simulink model "Simulations"  (R2020b)
settings: Solver=VariableStepAuto  StartTime=0.0  StopTime=100  MinStep=0.0001  RelTol=1e-3
undefined symbols (not defined in the file or in its folder): chassis, FTP, powertrain, sigbuilder_block
libraries: sdl_lib x364, nesl_utility x336, fl_lib x224, aerolibconvert2 x28, pid_lib x27
(part 1 of 15)
settings Model: Creator=moizk  LastModifiedBy=prshe

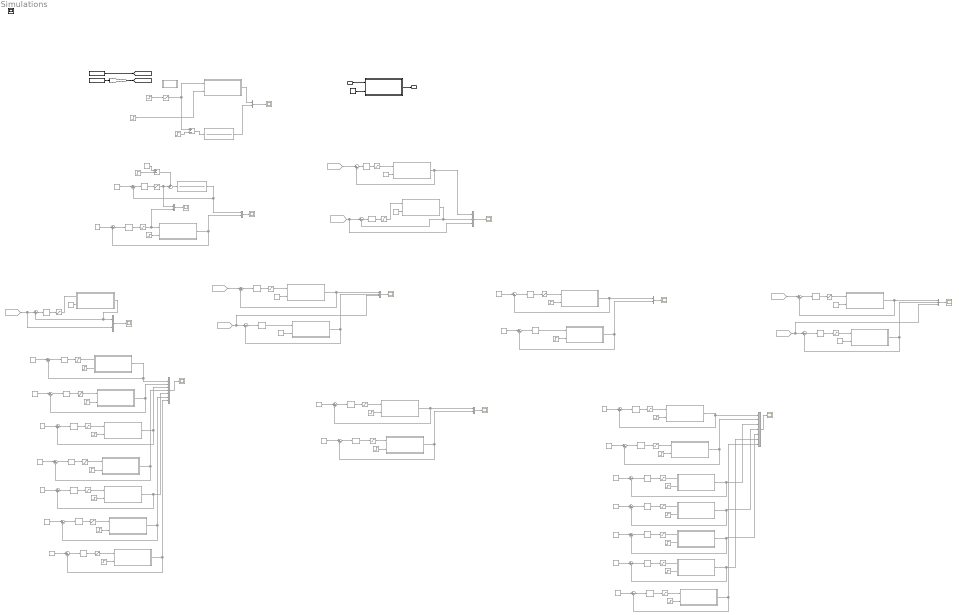
== system Simulations ==
  note: Non linear vs linear for constant speed
  note: System to linearize at a set point of 10 m/s
  note: Effect of motor delay removal on FTP
  note: Saturation block effects on FTP cycle
  note: Response to FTP
  note: Response to different hill slopes
  note: Vehicle Model
  note: Workspace (Import FTP drive cycle)
  note: Anti windup effects on constant speed with disturbance
  note: Saturation block effects on constant speed with disturbance
  note: Effects of different vehicle mass
  note: Effects of different vehicle mass for FTP
  torque : Inport
  Constant{,3..5,15..18} (8 alike) : Constant  Commented=on  Value=0
  Constant{1..2,7..14,19..28} (20 alike) : Constant  Commented=on  Value=10
  Constant6 : Constant  Value=0
  From{,1..6} (7 alike) : From  Commented=on  GotoTag=sch_cycle
  Motor removed : Subsystem  Commented=on
  Mux{,1..3,7..8} (6 alike) : Mux  Commented=on  Inputs=2
  Mux10 : Mux  Commented=on  Inputs=3
  Mux4 : Mux  Commented=on  Inputs=3
  Mux5 : Mux  Commented=on  Inputs=3
  Mux6 : Mux  Commented=on  Inputs=7
  Mux9 : Mux  Commented=on  Inputs=7
  PID Controller{1..10,12..27} (26 alike) : pid_lib/PID Controller  Commented=on  Controller=PID  Form=Parallel  TimeDomain=Continuous-time  UseExternalTs=off  SampleTime=-1  IntegratorMethod=Forward Euler  FilterMethod=Forward Euler  ControllerParametersSource=internal  P=0.8101  I=0.2270  D=0.2498  UseFilter=on  N=1000  TunerSelectOption=Transfer Function Based (PID Tuner App)  InitialConditionSource=internal  InitialConditionForIntegrator=0  InitialConditionForFilter=0  DifferentiatorICPrevScaledInput=0  ExternalReset=none  TrackingMode=off  Kt=1  LimitOutput=on  SatLimitsSource=internal  UpperSaturationLimit=powertrain.UpperTorqueLim  LowerSaturationLimit=powertrain.LowerTorqueLim  LinearizeAsGain=on  AntiWindupMode=back-calculation  Kb=0.3  POutMin=[]  POutMax=[]  IOutMin=[]  IOutMax=[]  DOutMin=[]  DOutMax=[]  NOutMin=[]  NOutMax=[]  SumOutMin=[]  SumOutMax=[]  SaturationOutMin=[]  SaturationOutMax=[]  PParamMin=[]  PParamMax=[]  IParamMin=[]  IParamMax=[]  DParamMin=[]  DParamMax=[]  NParamMin=[]  NParamMax=[]  KbParamMin=[]  KbParamMax=[]  KtParamMin=[]  KtParamMax=[]  KbOutMin=[]  KbOutMax=[]  KtOutMin=[]  KtOutMax=[]  IntegratorOutMin=[]  IntegratorOutMax=[]  FilterOutMin=[]  FilterOutMax=[]  SumI1OutMin=[]  SumI1OutMax=[]  SumI2OutMin=[]  SumI2OutMax=[]  SumI3OutMin=[]  SumI3OutMax=[]  SumI4OutMin=[]  SumI4OutMax=[]  SumDOutMin=[]  SumDOutMax=[]  DifferentiatorOutMin=[]  DifferentiatorOutMax=[]  FilterDiffOutCoefMin=[]  FilterDiffOutCoefMax=[]  ReciprocalOutMin=[]  ReciprocalOutMax=[]  SumDenOutMin=[]  SumDenOutMax=[]  SumNumOutMin=[]  SumNumOutMax=[]  DivideOutMin=[]  DivideOutMax=[]  UdiffTsProdOutMin=[]  UdiffTsProdOutMax=[]  NTsProdOutMin=[]  NTsProdOutMax=[]  UintegralTsProdOutMin=[]  UintegralTsProdOutMax=[]  UngainTsProdOutMin=[]  UngainTsProdOutMax=[]  IntegratorContinuousStateAttributes=''  IntegratorStateMustResolveToSignalObject=off  IntegratorRTWStateStorageClass=Auto  FilterContinuousStateAttributes=''  FilterStateMustResolveToSignalObject=off  FilterRTWStateStorageClass=Auto  ParallelPVariant=InternalParameters  IdealPVariant=Disabled  IVariant=InternalParameters  DVariant=InternalParameters  IntegratorVariant=Continuous  SatVariant=Enabled  AWVariant=BackCalculation  PCopyVariant=Disabled  TRVariant=Disabled  FdbkBlocksVariant=Forward  IdealPFdbkVariant=Disabled  SatFdbkVariant=Disabled  DerivativeFilterVariant=ContFilter  NVariant=InternalParameters  NCopyVariant=Disabled  FilterICVariant=InternalICsFilter  IntegratorICVariant=InternalICs  ExternalResetVariant=Disabled  TRSumVariant=Passthrough  SumFdbkVariant=Disabled  SumVariant=Sum_PID  TsampFilterVariant=InternalTs  TsampNgainVariant=Passthrough  TsampIntegralVariant=Passthrough  ExternalSaturationOutDataTypeStr=Inherit: Same as second input
  PID Controller11 : pid_lib/PID Controller  Commented=on  Controller=PID  Form=Parallel  TimeDomain=Continuous-time  UseExternalTs=off  SampleTime=-1  IntegratorMethod=Forward Euler  FilterMethod=Forward Euler  ControllerParametersSource=internal  P=0.8101  I=0.2270  D=0.2498  UseFilter=on  N=1000  TunerSelectOption=Transfer Function Based (PID Tuner App)  InitialConditionSource=internal  InitialConditionForIntegrator=0  InitialConditionForFilter=0  DifferentiatorICPrevScaledInput=0  ExternalReset=none  TrackingMode=off  Kt=1  LimitOutput=off  SatLimitsSource=internal  UpperSaturationLimit=powertrain.UpperTorqueLim  LowerSaturationLimit=powertrain.LowerTorqueLim  LinearizeAsGain=on  AntiWindupMode=back-calculation  Kb=0.3  POutMin=[]  POutMax=[]  IOutMin=[]  IOutMax=[]  DOutMin=[]  DOutMax=[]  NOutMin=[]  NOutMax=[]  SumOutMin=[]  SumOutMax=[]  SaturationOutMin=[]  SaturationOutMax=[]  PParamMin=[]  PParamMax=[]  IParamMin=[]  IParamMax=[]  DParamMin=[]  DParamMax=[]  NParamMin=[]  NParamMax=[]  KbParamMin=[]  KbParamMax=[]  KtParamMin=[]  KtParamMax=[]  KbOutMin=[]  KbOutMax=[]  KtOutMin=[]  KtOutMax=[]  IntegratorOutMin=[]  IntegratorOutMax=[]  FilterOutMin=[]  FilterOutMax=[]  SumI1OutMin=[]  SumI1OutMax=[]  SumI2OutMin=[]  SumI2OutMax=[]  SumI3OutMin=[]  SumI3OutMax=[]  SumI4OutMin=[]  SumI4OutMax=[]  SumDOutMin=[]  SumDOutMax=[]  DifferentiatorOutMin=[]  DifferentiatorOutMax=[]  FilterDiffOutCoefMin=[]  FilterDiffOutCoefMax=[]  ReciprocalOutMin=[]  ReciprocalOutMax=[]  SumDenOutMin=[]  SumDenOutMax=[]  SumNumOutMin=[]  SumNumOutMax=[]  DivideOutMin=[]  DivideOutMax=[]  UdiffTsProdOutMin=[]  UdiffTsProdOutMax=[]  NTsProdOutMin=[]  NTsProdOutMax=[]  UintegralTsProdOutMin=[]  UintegralTsProdOutMax=[]  UngainTsProdOutMin=[]  UngainTsProdOutMax=[]  IntegratorContinuousStateAttributes=''  IntegratorStateMustResolveToSignalObject=off  IntegratorRTWStateStorageClass=Auto  FilterContinuousStateAttributes=''  FilterStateMustResolveToSignalObject=off  FilterRTWStateStorageClass=Auto  ParallelPVariant=InternalParameters  IdealPVariant=Disabled  IVariant=InternalParameters  DVariant=InternalParameters  IntegratorVariant=Continuous  SatVariant=Disabled  AWVariant=Passthrough  PCopyVariant=Disabled  TRVariant=Disabled  FdbkBlocksVariant=Forward  IdealPFdbkVariant=Disabled  SatFdbkVariant=Disabled  DerivativeFilterVariant=ContFilter  NVariant=InternalParameters  NCopyVariant=Disabled  FilterICVariant=InternalICsFilter  IntegratorICVariant=InternalICs  ExternalResetVariant=Disabled  TRSumVariant=Passthrough  SumFdbkVariant=Disabled  SumVariant=Sum_PID  TsampFilterVariant=InternalTs  TsampNgainVariant=Passthrough  TsampIntegralVariant=Passthrough  ExternalSaturationOutDataTypeStr=Inherit: Same as second input
  Plant Model : Subsystem  Commented=on
  Plant Model1 : Subsystem
  Plant Model10 : Subsystem  Commented=on
  Plant Model11 : Subsystem  Commented=on
  Plant Model12 : Subsystem  Commented=on
  Plant Model13 : Subsystem  Commented=on
  Plant Model14 : Subsystem  Commented=on
  Plant Model15 : Subsystem  Commented=on
  Plant Model16 : Subsystem  Commented=on
  Plant Model17 : Subsystem  Commented=on
  Plant Model18 : Subsystem  Commented=on
  Plant Model19 : Subsystem  Commented=on
  Plant Model2 : Subsystem  Commented=on
  Plant Model20 : Subsystem  Commented=on
  Plant Model21 : Subsystem  Commented=on
  Plant Model22 : Subsystem  Commented=on
  Plant Model23 : Subsystem  Commented=on
  Plant Model24 : Subsystem  Commented=on
  Plant Model25 : Subsystem  Commented=on
  Plant Model26 : Subsystem  Commented=on
  Plant Model3 : Subsystem  Commented=on
  Plant Model4 : Subsystem  Commented=on
  Plant Model5 : Subsystem  Commented=on
  Plant Model6 : Subsystem  Commented=on
  Plant Model7 : Subsystem  Commented=on
  Plant Model8 : Subsystem  Commented=on
  Plant Model9 : Subsystem  Commented=on
  Saturation{1..26} (26 alike) : Saturate  Commented=on  UpperLimit=powertrain.UpperTorqueLim  LowerLimit=powertrain.LowerTorqueLim
  Scale Trace Spd : Gain  Gain=FTP.ScaledSpd
  Scope{,3..4,7..14} (11 alike) : Scope  Commented=on
  Step : Step  Commented=on  After=0.6484  SampleTime=0
  Step{1,3,5..6,8..12,18..22} (14 alike) : Step  Commented=on  Time=50  After=4  SampleTime=0
  Step13 : Step  Commented=on  Time=50  After=6  SampleTime=0
  Step14 : Step  Commented=on  Time=50  After=7  SampleTime=0
  Step15 : Step  Commented=on  Time=50  After=8  SampleTime=0
  Step16 : Step  Commented=on  Time=50  After=9  SampleTime=0
  Step17 : Step  Commented=on  Time=50  After=10  SampleTime=0
  Step2 : Step  Commented=on  Time=50  After=0.1987  SampleTime=0
  Step4 : Step  Commented=on  Time=50  After=0.1987  SampleTime=0
  Step7 : Step  Commented=on  Time=50  After=5  SampleTime=0
  Subtract : Sum  Commented=on  Inputs=+-
  Subtract1 : Sum  Commented=on  Inputs=+-
  Sum{,2..27} (27 alike) : Sum  Commented=on  Inputs=|+-
  Sum1 : Sum  Commented=on  Inputs=++|
  Transfer Fcn : TransferFcn  Commented=on  Numerator=[67.24]  Denominator=[1 12.22 22.63 4.36]
  Transfer Fcn2 : TransferFcn  Commented=on  Numerator=[67.24]  Denominator=[1 12.22 22.63 4.36]
  WrkSp Road Slope (Zero) : FromWorkspace  VariableName=FTP.sch_grade.data
  Wrksp Drive Cycle : FromWorkspace  VariableName=FTP.sch_cycle.data
  trq_cmd4 : Subsystem  Tag=STV Subsys  Commented=on  LoadFcn=sigbuilder_block('load');  StartFcn=sigbuilder_block('start');  StopFcn=sigbuilder_block('stop');  ClipboardFcn=sigbuilder_block('clipboard');  mask(Sigbuilder block){tuvar=[0:10]}
      mask help: Simulink:masks:SigbuilderBlock_MD
      mask init:
      | if ~strcmp(get_param(bdroot(gcbh),'SimulationStatus'),'stopped') tuvar = sigbuilder_block('maskInit'); end
      settings: CopyFcn=sigbuilder_block('copy');  DeleteFcn=sigbuilder_block('delete');  ModelCloseFcn=sigbuilder_block('modelClose');  PreSaveFcn=sigbuilder_block('preSave');  PauseFcn=sigbuilder_block('pause');  ContinueFcn=sigbuilder_block('continue');  NameChangeFcn=sigbuilder_block('namechange');  OpenFcn=sigbuilder_block('open',[0 30 1152 561.6 ]);  CloseFcn=sigbuilder_block('close');
      mask Display: plot(0, 0, 100, 100,[2, 2, 32, 32, 2], [68, 8, 8, 68, 68],[32, 2], [38, 38], [32, 19, 2],[53, 60, 44], [32, 17, 17, 2],[16, 16, 31, 31]);txt = getActiveGroup(gcbh);text(2, 100, txt,'verticalAlignment', 'top');
  speed : Outport
  Scope{1..2,5..6} (4 alike) : Scope
  wires:
  WrkSp Road Slope (Zero)/1 -> [sch_grade]
  Step1/1 -> Plant Model/2(road_grade)
  Plant Model/1(veh_spd_lin) -> Mux/1  "Model Velo (m/s)"
  Wrksp Drive Cycle/1 -> Scale Trace Spd/1
  Scale Trace Spd/1 -> [sch_cycle]
  Step/1 -> Saturation1/1  "trq_cmd"
  Saturation1/1 -> Subtract/1, Plant Model/1(trq_cmd)  "trq_act"
  Mux/1 -> Scope/1
  Transfer Fcn/1 -> Mux/2
  Step2/1 -> Subtract/2
  Subtract/1 -> Transfer Fcn/1
  Plant Model3/1(veh_spd_lin) -> Mux1/1, Sum/2  "Output Speed"
  Sum/1 -> PID Controller2/1
  From/1 -> Mux1/2, Sum/1  "Desired Speed"
  Step4/1 -> Subtract1/2
  Constant/1 -> Subtract1/1
  PID Controller2/1 -> Saturation2/1
  Saturation2/1 -> Plant Model3/1(trq_cmd)
  Mux1/1 -> Scope3/1
  Sum1/1 -> Transfer Fcn2/1
  Transfer Fcn2/1 -> Mux2/1, Sum2/2  "Linear"
  PID Controller10/1 -> Saturation3/1  "before sat"
  Saturation3/1 -> Mux3/1, Sum1/2  "torque-linear"
  Subtract1/1 -> Sum1/1
  Constant2/1 -> Sum2/1
  Sum2/1 -> PID Controller10/1
  Constant6/1 -> Plant Model1/2(road_grade)
  torque/1 -> Plant Model1/1(trq_cmd)
  Plant Model1/1(veh_spd_lin) -> speed/1
  PID Controller1/1 -> Saturation4/1
  Sum4/1 -> PID Controller1/1
  Plant Model2/1(veh_spd_lin) -> Mux2/2, Sum4/2  "Nonlinear"
  Constant1/1 -> Sum4/1
  Saturation4/1 -> Mux3/2, Plant Model2/1(trq_cmd)  "torque-nonlinear"
  Step6/1 -> Plant Model2/2(road_grade)
  Mux2/1 -> Scope4/1
  Mux3/1 -> Scope7/1
  Constant3/1 -> Plant Model3/2(road_grade)
  Constant4/1 -> Plant Model4/2(road_grade)
  PID Controller4/1 -> Saturation5/1
  Saturation5/1 -> Plant Model4/1(trq_cmd)
  Mux4/1 -> Scope8/1
  Plant Model4/1(veh_spd_lin) -> Sum3/2, Mux4/2  "Control"
  Sum3/1 -> PID Controller4/1
  From1/1 -> Mux4/3, Sum3/1  "Desired Speed"
  From2/1 -> Sum5/1  "Desired Speed"
  Sum5/1 -> PID Controller3/1
  PID Controller3/1 -> Saturation6/1
  Saturation6/1 -> Motor removed/1(trq_cmd)
  Constant5/1 -> Motor removed/2(road_grade)
  Motor removed/1(veh_spd_lin) -> Mux4/1, Sum5/2  "Motor removed"
  From3/1 -> Sum6/1
  Constant15/1 -> Plant Model5/2(road_grade)
  Plant Model5/1(veh_spd_lin) -> Mux5/1, Sum6/2  "Saturation"
  PID Controller5/1 -> Saturation7/1
  Sum6/1 -> PID Controller5/1
  Saturation7/1 -> Plant Model5/1(trq_cmd)  "torque-nonlinear"
  From4/1 -> Mux5/3, Sum7/1  "Desired Speed"
  Constant16/1 -> Plant Model6/2(road_grade)
  Plant Model6/1(veh_spd_lin) -> Mux5/2, Sum7/2  "No saturation"
  Sum7/1 -> PID Controller6/1
  PID Controller6/1 -> Plant Model6/1(trq_cmd)  "torque-nonlinear"
  Mux5/1 -> Scope9/1
  Constant9/1 -> Sum8/1
  Step7/1 -> Plant Model7/2(road_grade)
  Plant Model7/1(veh_spd_lin) -> Mux6/2, Sum8/2  "5 degrees"
  PID Controller8/1 -> Saturation8/1
  Sum8/1 -> PID Controller8/1
  Saturation8/1 -> Plant Model7/1(trq_cmd)  "torque-nonlinear"
  Sum9/1 -> PID Controller7/1
  Plant Model8/1(veh_spd_lin) -> Mux6/1, Sum9/2  "4 degrees"
  Step8/1 -> Plant Model8/2(road_grade)
  PID Controller7/1 -> Saturation9/1
  Saturation9/1 -> Plant Model8/1(trq_cmd)  "torque-nonlinear"
  Constant10/1 -> Sum9/1
  Mux6/1 -> Scope10/1
  Mux7/1 -> Scope11/1
  Saturation10/1 -> Plant Model9/1(trq_cmd)  "torque-nonlinear"
  Plant Model9/1(veh_spd_lin) -> Mux7/1, Sum10/2  "With anti-windup"
  Step9/1 -> Plant Model9/2(road_grade)
  Constant11/1 -> Sum10/1
  Sum10/1 -> PID Controller9/1
  PID Controller11/1 -> Saturation11/1  "torque-nonlinear"
  Sum11/1 -> PID Controller11/1
  PID Controller9/1 -> Saturation10/1
  Plant Model10/1(veh_spd_lin) -> Mux7/2, Sum11/2  "No anti-windup"
  Constant12/1 -> Sum11/1
  Step10/1 -> Plant Model10/2(road_grade)
  Saturation11/1 -> Plant Model10/1(trq_cmd)  "torque-nonlinear"
  Mux8/1 -> Scope12/1
  Saturation12/1 -> Plant Model11/1(trq_cmd)  "torque-nonlinear"
  Plant Model11/1(veh_spd_lin) -> Mux8/1, Sum12/2  "Saturation"
  Step11/1 -> Plant Model11/2(road_grade)
  Constant13/1 -> Sum12/1
  Sum12/1 -> PID Controller12/1
  PID Controller13/1 -> Plant Model12/1(trq_cmd)  "torque-nonlinear"
  Sum13/1 -> PID Controller13/1
  PID Controller12/1 -> Saturation12/1
  Plant Model12/1(veh_spd_lin) -> Mux8/2, Sum13/2  "No saturation"
  Constant14/1 -> Sum13/1
  Step12/1 -> Plant Model12/2(road_grade)
  Sum15/1 -> PID Controller15/1
  Constant8/1 -> Sum15/1
  Plant Model14/1(veh_spd_lin) -> Sum15/2, Mux9/2  "5kg"
  Step5/1 -> Plant Model14/2(road_grade)
  PID Controller14/1 -> Saturation13/1
  Sum14/1 -> PID Controller14/1
  PID Controller15/1 -> Saturation14/1  "torque-nonlinear"
  Constant7/1 -> Sum14/1
  Mux9/1 -> Scope13/1
  Plant Model13/1(veh_spd_lin) -> Sum14/2, Mux9/1  "4.84kg"
  Saturation13/1 -> Plant Model13/1(trq_cmd)  "torque-nonlinear"
  Step3/1 -> Plant Model13/2(road_grade)
  Saturation14/1 -> Plant Model14/1(trq_cmd)  "torque-nonlinear"
  Sum16/1 -> PID Controller16/1
  Saturation16/1 -> Plant Model16/1(trq_cmd)  "torque-nonlinear"
  PID Controller16/1 -> Saturation15/1
  PID Controller17/1 -> Saturation16/1  "torque-nonlinear"
  Constant18/1 -> Plant Model16/2(road_grade)
  Plant Model16/1(veh_spd_lin) -> Mux10/2, Sum17/2  "6kg"
  From5/1 -> Sum16/1
  Sum17/1 -> PID Controller17/1
  Mux10/1 -> Scope14/1
  Plant Model15/1(veh_spd_lin) -> Mux10/1, Sum16/2  "4.84kg"
  Constant17/1 -> Plant Model15/2(road_grade)
  Saturation15/1 -> Plant Model15/1(trq_cmd)  "torque-nonlinear"
  From6/1 -> Mux10/3, Sum17/1  "Desired speed"
  PID Controller18/1 -> Saturation17/1
  Plant Model17/1(veh_spd_lin) -> Mux6/3, Sum18/2  "6 degrees"
  Sum18/1 -> PID Controller18/1
  Step13/1 -> Plant Model17/2(road_grade)
  Constant19/1 -> Sum18/1
  Saturation17/1 -> Plant Model17/1(trq_cmd)  "torque-nonlinear"
  PID Controller19/1 -> Saturation18/1
  Plant Model18/1(veh_spd_lin) -> Mux6/4, Sum19/2  "7 degrees"
  Sum19/1 -> PID Controller19/1
  Step14/1 -> Plant Model18/2(road_grade)
  Constant20/1 -> Sum19/1
  Saturation18/1 -> Plant Model18/1(trq_cmd)  "torque-nonlinear"
  PID Controller20/1 -> Saturation19/1
  Plant Model19/1(veh_spd_lin) -> Mux6/5, Sum20/2  "8 degrees"
  Sum20/1 -> PID Controller20/1
  Step15/1 -> Plant Model19/2(road_grade)
  Constant21/1 -> Sum20/1
  Saturation19/1 -> Plant Model19/1(trq_cmd)  "torque-nonlinear"
  PID Controller21/1 -> Saturation20/1
  Plant Model20/1(veh_spd_lin) -> Mux6/6, Sum21/2  "9 degrees"
  Sum21/1 -> PID Controller21/1
  Step16/1 -> Plant Model20/2(road_grade)
  Constant22/1 -> Sum21/1
  Saturation20/1 -> Plant Model20/1(trq_cmd)  "torque-nonlinear"
  PID Controller22/1 -> Saturation21/1
  Plant Model21/1(veh_spd_lin) -> Mux6/7, Sum22/2  "10 degrees"
  Sum22/1 -> PID Controller22/1
  Step17/1 -> Plant Model21/2(road_grade)
  Constant23/1 -> Sum22/1
  Saturation21/1 -> Plant Model21/1(trq_cmd)  "torque-nonlinear"
  Plant Model22/1(veh_spd_lin) -> Mux9/3, Sum23/2  "6kg"
  Saturation22/1 -> Plant Model22/1(trq_cmd)  "torque-nonlinear"
  Sum23/1 -> PID Controller23/1
  Constant24/1 -> Sum23/1
  Step18/1 -> Plant Model22/2(road_grade)
  PID Controller23/1 -> Saturation22/1  "torque-nonlinear"
  Plant Model23/1(veh_spd_lin) -> Mux9/4, Sum24/2  "7kg"
  Saturation23/1 -> Plant Model23/1(trq_cmd)  "torque-nonlinear"
  Sum24/1 -> PID Controller24/1
  Constant25/1 -> Sum24/1
  Step19/1 -> Plant Model23/2(road_grade)
  PID Controller24/1 -> Saturation23/1  "torque-nonlinear"
  Plant Model24/1(veh_spd_lin) -> Mux9/5, Sum25/2  "8kg"
  Saturation24/1 -> Plant Model24/1(trq_cmd)  "torque-nonlinear"
  Sum25/1 -> PID Controller25/1
  Constant26/1 -> Sum25/1
  Step20/1 -> Plant Model24/2(road_grade)
  PID Controller25/1 -> Saturation24/1  "torque-nonlinear"
  Plant Model25/1(veh_spd_lin) -> Mux9/6, Sum26/2  "9kg"
  Saturation25/1 -> Plant Model25/1(trq_cmd)  "torque-nonlinear"
  Sum26/1 -> PID Controller26/1
  Constant27/1 -> Sum26/1
  Step21/1 -> Plant Model25/2(road_grade)
  PID Controller26/1 -> Saturation25/1  "torque-nonlinear"
  Plant Model26/1(veh_spd_lin) -> Mux9/7, Sum27/2  "10kg"
  Saturation26/1 -> Plant Model26/1(trq_cmd)  "torque-nonlinear"
  Sum27/1 -> PID Controller27/1
  Constant28/1 -> Sum27/1
  Step22/1 -> Plant Model26/2(road_grade)
  PID Controller27/1 -> Saturation26/1  "torque-nonlinear"

== system Simulations/Motor removed ==
  note: Chassis
  note: Motor Dynamics
  note: Drivetrain
  trq_cmd : Inport
  road_grade : Inport  Port=2
  Angle Conversion3 : aerolibconvert2/Angle Conversion  IU=deg  OU=rad
  Belt Drive FL : sdl_lib/Couplings & Drives/Belt Drive  drive_type=sdl.enum.wrap_configuration.open  belt_type=sdl.enum.belt_type.ideal  sheave_ang=30 deg  num_belts=1  model_f_c=sdl.enum.model_centrifugal.off  linear_density=0.6 kg/m  model_compliance=sdl.enum.compliance.off  stiffness=1e4 N/m  damping=1e3 N/(m/s)  tension=100 N  breakable=sdl.enum.max_tension.off  F_max=1e5 N  r_pulley_A=drivetrain.RadiusA m  r_pulley_B=drivetrain.RadiusB m  b_pulley_A=drivetrain.bvfCoeffA N*m/(rad/s)  b_pulley_B=drivetrain.bvfCoeffB N*m/(rad/s)  model_inertia_A=sdl.enum.model_inertia.off  model_inertia_B=sdl.enum.model_inertia.off  pulley_inertia_A=0.01 kg*m^2  pulley_inertia_B=0.03 kg*m^2  initial_velocity_A=0 rad/s  initial_velocity_B=0 rad/s  mu=0.5  wrap_parameterization=sdl.enum.wrap_parameterization.centers  d_centers=0.5 m  phi_wrap_A=145 deg  phi_wrap_B=215 deg  v_thr=0.001 m/s
      settings: SourceProductBaseCode=LD  InternalSimscapePortConfiguration="{\"Bottom\":[],\"Left\":[{\"id\":\"A\",\"label\":\"A\",\"type\":\"foundation.mechanical.rotational.rotational\"}],\"Right\":[{\"id\":\"B\",\"label\":\"B\",\"type\":\"foundation.mechanical.rotational.rotational\"}],\"Top\":[]}"
  Belt Drive FR : sdl_lib/Couplings & Drives/Belt Drive  drive_type=sdl.enum.wrap_configuration.open  belt_type=sdl.enum.belt_type.ideal  sheave_ang=30 deg  num_belts=1  model_f_c=sdl.enum.model_centrifugal.off  linear_density=0.6 kg/m  model_compliance=sdl.enum.compliance.off  stiffness=1e4 N/m  damping=1e3 N/(m/s)  tension=100 N  breakable=sdl.enum.max_tension.off  F_max=1e5 N  r_pulley_A=drivetrain.RadiusA m  r_pulley_B=drivetrain.RadiusB m  b_pulley_A=drivetrain.bvfCoeffA N*m/(rad/s)  b_pulley_B=drivetrain.bvfCoeffB N*m/(rad/s)  model_inertia_A=sdl.enum.model_inertia.off  model_inertia_B=sdl.enum.model_inertia.off  pulley_inertia_A=0.01 kg*m^2  pulley_inertia_B=0.03 kg*m^2  initial_velocity_A=0 rad/s  initial_velocity_B=0 rad/s  mu=0.5  wrap_parameterization=sdl.enum.wrap_parameterization.centers  d_centers=0.5 m  phi_wrap_A=145 deg  phi_wrap_B=215 deg  v_thr=0.001 m/s
      settings: SourceProductBaseCode=LD  InternalSimscapePortConfiguration="{\"Bottom\":[],\"Left\":[{\"id\":\"A\",\"label\":\"A\",\"type\":\"foundation.mechanical.rotational.rotational\"}],\"Right\":[{\"id\":\"B\",\"label\":\"B\",\"type\":\"foundation.mechanical.rotational.rotational\"}],\"Top\":[]}"
  Belt Drive RL : sdl_lib/Couplings & Drives/Belt Drive  drive_type=sdl.enum.wrap_configuration.open  belt_type=sdl.enum.belt_type.ideal  sheave_ang=30 deg  num_belts=1  model_f_c=sdl.enum.model_centrifugal.off  linear_density=0.6 kg/m  model_compliance=sdl.enum.compliance.off  stiffness=1e4 N/m  damping=1e3 N/(m/s)  tension=100 N  breakable=sdl.enum.max_tension.off  F_max=1e5 N  r_pulley_A=drivetrain.RadiusA m  r_pulley_B=drivetrain.RadiusB m  b_pulley_A=drivetrain.bvfCoeffA N*m/(rad/s)  b_pulley_B=drivetrain.bvfCoeffB N*m/(rad/s)  model_inertia_A=sdl.enum.model_inertia.off  model_inertia_B=sdl.enum.model_inertia.off  pulley_inertia_A=0.01 kg*m^2  pulley_inertia_B=0.03 kg*m^2  initial_velocity_A=0 rad/s  initial_velocity_B=0 rad/s  mu=0.5  wrap_parameterization=sdl.enum.wrap_parameterization.centers  d_centers=0.5 m  phi_wrap_A=145 deg  phi_wrap_B=215 deg  v_thr=0.001 m/s
      settings: SourceProductBaseCode=LD  InternalSimscapePortConfiguration="{\"Bottom\":[],\"Left\":[{\"id\":\"A\",\"label\":\"A\",\"type\":\"foundation.mechanical.rotational.rotational\"}],\"Right\":[{\"id\":\"B\",\"label\":\"B\",\"type\":\"foundation.mechanical.rotational.rotational\"}],\"Top\":[]}"
  Belt Drive RR : sdl_lib/Couplings & Drives/Belt Drive  drive_type=sdl.enum.wrap_configuration.open  belt_type=sdl.enum.belt_type.ideal  sheave_ang=30 deg  num_belts=1  model_f_c=sdl.enum.model_centrifugal.off  linear_density=0.6 kg/m  model_compliance=sdl.enum.compliance.off  stiffness=1e4 N/m  damping=1e3 N/(m/s)  tension=100 N  breakable=sdl.enum.max_tension.off  F_max=1e5 N  r_pulley_A=drivetrain.RadiusA m  r_pulley_B=drivetrain.RadiusB m  b_pulley_A=drivetrain.bvfCoeffA N*m/(rad/s)  b_pulley_B=drivetrain.bvfCoeffB N*m/(rad/s)  model_inertia_A=sdl.enum.model_inertia.off  model_inertia_B=sdl.enum.model_inertia.off  pulley_inertia_A=0.01 kg*m^2  pulley_inertia_B=0.03 kg*m^2  initial_velocity_A=0 rad/s  initial_velocity_B=0 rad/s  mu=0.5  wrap_parameterization=sdl.enum.wrap_parameterization.centers  d_centers=0.5 m  phi_wrap_A=145 deg  phi_wrap_B=215 deg  v_thr=0.001 m/s
      settings: SourceProductBaseCode=LD  InternalSimscapePortConfiguration="{\"Bottom\":[],\"Left\":[{\"id\":\"A\",\"label\":\"A\",\"type\":\"foundation.mechanical.rotational.rotational\"}],\"Right\":[{\"id\":\"B\",\"label\":\"B\",\"type\":\"foundation.mechanical.rotational.rotational\"}],\"Top\":[]}"
  Constant : Constant  Value=0
  Ideal Torque Source FL : fl_lib/Mechanical/Mechanical Sources/Ideal Torque Source
  Ideal Torque Source FR : fl_lib/Mechanical/Mechanical Sources/Ideal Torque Source
  Ideal Torque Source RL : fl_lib/Mechanical/Mechanical Sources/Ideal Torque Source
  Ideal Torque Source RR : fl_lib/Mechanical/Mechanical Sources/Ideal Torque Source
  Mechanical Rotational Reference{1..3,8} (4 alike) : fl_lib/Mechanical/Rotational Elements/Mechanical Rotational Reference
  PS-Simulink Converter{,1,3..4} (4 alike) : nesl_utility/PS-Simulink Converter  PhysicalDomain=network_engine_domain  SubClassName=ps_output  LeftPortType=input  RightPortType=output  PseudoPeriodic=off  Frequencies=[]  Unit=inherit  AffineConversion=off
  Simulink-PS Converter{3,9..12} (5 alike) : nesl_utility/Simulink-PS Converter  PhysicalDomain=network_engine_domain  SubClassName=ps_input  LeftPortType=input  RightPortType=output  PseudoPeriodic=off  Frequencies=[]  NoiseDistribution=none  NoiseParameters=[]  Unit=1  AffineConversion=off  FilteringAndDerivatives=provide  SimscapeFilterOrder=1  InputFilterTimeConstant=0.001  UdotUserProvided=0
  Simulink-PS Converter8 : nesl_utility/Simulink-PS Converter  PhysicalDomain=network_engine_domain  SubClassName=ps_input  LeftPortType=input  RightPortType=output  PseudoPeriodic=off  Frequencies=[]  NoiseDistribution=none  NoiseParameters=[]  Unit=rad  AffineConversion=off  FilteringAndDerivatives=provide  SimscapeFilterOrder=1  InputFilterTimeConstant=0.001  UdotUserProvided=0
  Solver Configuration2 : nesl_utility/Solver Configuration  PhysicalDomain=network_engine_domain  SubClassName=solver  LeftPortType=input  RightPortType=generic  Tones=[]  Harmonics=[]  SimulateNoise=off  Profile=off  UseLocalSampling=off  EnableSwitchedLinearOptims=on  FrequencyDomain=off  UseCCode=off  RelTol=0.001  AbsTol=1e-06  MinStep=1e-09  ToWorkspace=off  RevertToSquareIcSolve=off  NumHomotopyIterations=100  PhasorMode=off  PhasorModeNumHarmonics=1  DoDC=off  ResidualTolerance=1e-09  UseLocalSolver=off  LocalSolverChoice=NE_BACKWARD_EULER_ADVANCER  LocalSolverSampleTime=0.001  DoFixedCost=off  MaxNonlinIter=3  MaxModeIter=2  ComputeImpulses=off  ImpulseIterations=2  LinearAlgebra=auto  EquationFormulation=NE_TIME_EF  DelaysMemoryBudget=1024  AutomaticFiltering=on  FilteringTimeConstant=0.001  PartitionStorageMethod=AS_NEEDED  PartitionMemoryBudget=1024  PartitionMethod=ROBUST
  Terminator{,1..3} (4 alike) : Terminator
  Tire (Simple) FL : sdl_lib/Tires & Vehicles/Tire (Simple)  r_tire=drivetrain.RolRadius m  model_compliance=0  stiffness=1e6 N/m  damping=1000 N/(m/s)  model_inertia=0  tire_inertia=drivetrain.IyyWhl kg*m^2  initial_velocity=drivetrain.InitVelo rad/s
      settings: SourceProductBaseCode=LD  InternalSimscapePortConfiguration="{\"Bottom\":[],\"Left\":[{\"id\":\"A\",\"label\":\"A\",\"type\":\"foundation.mechanical.rotational.rotational\"}],\"Right\":[{\"id\":\"H\",\"label\":\"H\",\"type\":\"foundation.mechanical.translational.translational\"}],\"Top\":[]}"
  Tire (Simple) FR : sdl_lib/Tires & Vehicles/Tire (Simple)  r_tire=drivetrain.RolRadius m  model_compliance=0  stiffness=1e6 N/m  damping=1000 N/(m/s)  model_inertia=0  tire_inertia=drivetrain.IyyWhl kg*m^2  initial_velocity=drivetrain.InitVelo rad/s
      settings: SourceProductBaseCode=LD  InternalSimscapePortConfiguration="{\"Bottom\":[],\"Left\":[{\"id\":\"A\",\"label\":\"A\",\"type\":\"foundation.mechanical.rotational.rotational\"}],\"Right\":[{\"id\":\"H\",\"label\":\"H\",\"type\":\"foundation.mechanical.translational.translational\"}],\"Top\":[]}"
  Tire (Simple) RL : sdl_lib/Tires & Vehicles/Tire (Simple)  r_tire=drivetrain.RolRadius m  model_compliance=0  stiffness=1e6 N/m  damping=1000 N/(m/s)  model_inertia=0  tire_inertia=drivetrain.IyyWhl kg*m^2  initial_velocity=drivetrain.InitVelo rad/s
      settings: SourceProductBaseCode=LD  InternalSimscapePortConfiguration="{\"Bottom\":[],\"Left\":[{\"id\":\"A\",\"label\":\"A\",\"type\":\"foundation.mechanical.rotational.rotational\"}],\"Right\":[{\"id\":\"H\",\"label\":\"H\",\"type\":\"foundation.mechanical.translational.translational\"}],\"Top\":[]}"
  Tire (Simple) RR : sdl_lib/Tires & Vehicles/Tire (Simple)  r_tire=drivetrain.RolRadius m  model_compliance=0  stiffness=1e6 N/m  damping=1000 N/(m/s)  model_inertia=0  tire_inertia=drivetrain.IyyWhl kg*m^2  initial_velocity=drivetrain.InitVelo rad/s
      settings: SourceProductBaseCode=LD  InternalSimscapePortConfiguration="{\"Bottom\":[],\"Left\":[{\"id\":\"A\",\"label\":\"A\",\"type\":\"foundation.mechanical.rotational.rotational\"}],\"Right\":[{\"id\":\"H\",\"label\":\"H\",\"type\":\"foundation.mechanical.translational.translational\"}],\"Top\":[]}"
  Tire-Road Interaction (Magic Formula) FL : sdl_lib/Tires & Vehicles/Tire Subcomponents/Tire-Road Interaction (Magic Formula)  parameterization=sdl.enum.magic_tire_model.peak  F_z1=drivetrain.VertLoad N  F_x1=drivetrain.PeakLongF N  kappa1=drivetrain.Slip  B_m=10  C_m=1.9  D_m=1  E_m=0.97  fz0=4000 N  p_Cx=1.685  p_Dx=[1.21, -.037]  p_Ex=[.344, .095, -.02, 0]  p_Kx=[21.51, -.163, .245]  p_Hx=[-.002, .002]  p_Vx=[0, 0]  v_tr_thr=drivetrain.VeloTrhd m/s
      settings: SourceProductBaseCode=LD  InternalSimscapePortConfiguration="{\"Bottom\":[],\"Left\":[{\"id\":\"N\",\"label\":\"N\",\"type\":\"input\"},{\"id\":\"T\",\"label\":\"T\",\"type\":\"foundation.mechanical.translational.translational\"}],\"Right\":[{\"id\":\"S\",\"label\":\"S\",\"type\":\"output\"},{\"id\":\"H\",\"label\":\"H\",\"type\":\"foundation.mechanical.translational.translational\"}],\"Top\":[]}"
  Tire-Road Interaction (Magic Formula) FR : sdl_lib/Tires & Vehicles/Tire Subcomponents/Tire-Road Interaction (Magic Formula)  parameterization=sdl.enum.magic_tire_model.peak  F_z1=drivetrain.VertLoad N  F_x1=drivetrain.PeakLongF N  kappa1=drivetrain.Slip  B_m=10  C_m=1.9  D_m=1  E_m=0.97  fz0=4000 N  p_Cx=1.685  p_Dx=[1.21, -.037]  p_Ex=[.344, .095, -.02, 0]  p_Kx=[21.51, -.163, .245]  p_Hx=[-.002, .002]  p_Vx=[0, 0]  v_tr_thr=drivetrain.VeloTrhd m/s
      settings: SourceProductBaseCode=LD  InternalSimscapePortConfiguration="{\"Bottom\":[],\"Left\":[{\"id\":\"N\",\"label\":\"N\",\"type\":\"input\"},{\"id\":\"T\",\"label\":\"T\",\"type\":\"foundation.mechanical.translational.translational\"}],\"Right\":[{\"id\":\"S\",\"label\":\"S\",\"type\":\"output\"},{\"id\":\"H\",\"label\":\"H\",\"type\":\"foundation.mechanical.translational.translational\"}],\"Top\":[]}"
  Tire-Road Interaction (Magic Formula) RL : sdl_lib/Tires & Vehicles/Tire Subcomponents/Tire-Road Interaction (Magic Formula)  parameterization=sdl.enum.magic_tire_model.peak  F_z1=drivetrain.VertLoad N  F_x1=drivetrain.PeakLongF N  kappa1=drivetrain.Slip  B_m=10  C_m=1.9  D_m=1  E_m=0.97  fz0=4000 N  p_Cx=1.685  p_Dx=[1.21, -.037]  p_Ex=[.344, .095, -.02, 0]  p_Kx=[21.51, -.163, .245]  p_Hx=[-.002, .002]  p_Vx=[0, 0]  v_tr_thr=drivetrain.VeloTrhd m/s
      settings: SourceProductBaseCode=LD  InternalSimscapePortConfiguration="{\"Bottom\":[],\"Left\":[{\"id\":\"N\",\"label\":\"N\",\"type\":\"input\"},{\"id\":\"T\",\"label\":\"T\",\"type\":\"foundation.mechanical.translational.translational\"}],\"Right\":[{\"id\":\"S\",\"label\":\"S\",\"type\":\"output\"},{\"id\":\"H\",\"label\":\"H\",\"type\":\"foundation.mechanical.translational.translational\"}],\"Top\":[]}"
  Tire-Road Interaction (Magic Formula) RR : sdl_lib/Tires & Vehicles/Tire Subcomponents/Tire-Road Interaction (Magic Formula)  parameterization=sdl.enum.magic_tire_model.peak  F_z1=drivetrain.VertLoad N  F_x1=drivetrain.PeakLongF N  kappa1=drivetrain.Slip  B_m=10  C_m=1.9  D_m=1  E_m=0.97  fz0=4000 N  p_Cx=1.685  p_Dx=[1.21, -.037]  p_Ex=[.344, .095, -.02, 0]  p_Kx=[21.51, -.163, .245]  p_Hx=[-.002, .002]  p_Vx=[0, 0]  v_tr_thr=drivetrain.VeloTrhd m/s
      settings: SourceProductBaseCode=LD  InternalSimscapePortConfiguration="{\"Bottom\":[],\"Left\":[{\"id\":\"N\",\"label\":\"N\",\"type\":\"input\"},{\"id\":\"T\",\"label\":\"T\",\"type\":\"foundation.mechanical.translational.translational\"}],\"Right\":[{\"id\":\"S\",\"label\":\"S\",\"type\":\"output\"},{\"id\":\"H\",\"label\":\"H\",\"type\":\"foundation.mechanical.translational.translational\"}],\"Top\":[]}"
  Vehicle Body : sdl_lib/Tires & Vehicles/Vehicle Body  mass=chassis.m kg  n_w=chassis.NumWhl  x_f=chassis.a m  x_r=chassis.b m  y_c="chassis.h  m"  mass_var=simscape.enum.onoff.off  model_pitch=simscape.enum.onoff.off  inertia=4000 kg*m^2  suspension_model=sdl.enum.linearTLU.linear  k_f=1e4 N/m  b_f=1e4 N/(m/s)  k_r=1e4 N/m  b_r=1e4 N/(m/s)  k_f_TLU=[-2000, -1000, 0, 1000, 2000] N  x_f_TLU=[-.4, -.2, 0, .2, .4] m  b_f_TLU=[-200, -100, 0, 100, 200] N  v_f_TLU=[-4, -2, 0, 2, 4] m/s  k_r_TLU=[-2000, -1000, 0, 1000, 2000] N  x_r_TLU=[-.4, -.2, 0, .2, .4] m  b_r_TLU=[-200, -100, 0, 100, 200] N  v_r_TLU=[-4, -2, 0, 2, 4] m/s  interp_method=simscape.enum.interpolation.linear  extrap_method=simscape.enum.extrapolation.linear  model_hardstop=simscape.enum.onoff.off  upper_bound_f=.25 m  lower_bound_f=-.25 m  stop_k_f=1e6 N/m  stop_b_f=150 N/(m/s)  upper_bound_r=.25 m  lower_bound_r=-.25 m  stop_k_r=1e6 N/m  stop_b_r=150 N/(m/s)  initial_pitch=0 rad  initial_pitch_rate=0 rad/s  g=chassis.g m/s^2  liftoff_warning=simscape.enum.onoff.off  area=chassis.Af m^2  Cd=chassis.Cd  rho=chassis.AirDensity kg/m^3  v_specify=off  v_priority=High  v=0 m/s  v_nominal_specify=off  v_nominal_unit=m/s  v_nominal_value=1
  v_lin1 : nesl_utility/PS-Simulink Converter  PhysicalDomain=network_engine_domain  SubClassName=ps_output  LeftPortType=input  RightPortType=output  PseudoPeriodic=off  Frequencies=[]  Unit=inherit  AffineConversion=off
  veh_spd_lin : Outport
  wires:
  trq_cmd/1 -> Simulink-PS Converter9/1, Simulink-PS Converter11/1, Simulink-PS Converter12/1, Simulink-PS Converter10/1  "trq_act"
  v_lin1/1 -> veh_spd_lin/1  "act"
  PS-Simulink Converter/1 -> Terminator/1
  PS-Simulink Converter1/1 -> Terminator1/1
  PS-Simulink Converter3/1 -> Terminator2/1
  PS-Simulink Converter4/1 -> Terminator3/1
  road_grade/1 -> Angle Conversion3/1
  Angle Conversion3/1 -> Simulink-PS Converter8/1
  Constant/1 -> Simulink-PS Converter3/1
  connections:
  Vehicle Body/RConn2 -- Tire-Road Interaction (Magic Formula) FR/LConn1 -- Tire-Road Interaction (Magic Formula) FL/LConn1
  Vehicle Body/LConn1 -- Tire-Road Interaction (Magic Formula) RR/RConn2 -- Tire-Road Interaction (Magic Formula) RL/RConn2 -- Tire-Road Interaction (Magic Formula) FR/RConn2 -- Tire-Road Interaction (Magic Formula) FL/RConn2
  Solver Configuration2/RConn1 -- Simulink-PS Converter9/RConn1 -- Ideal Torque Source RR/RConn1
  Vehicle Body/RConn1 -- Tire-Road Interaction (Magic Formula) RR/LConn1 -- Tire-Road Interaction (Magic Formula) RL/LConn1
  Belt Drive FR/RConn1 -- Tire (Simple) FR/LConn1
  Simulink-PS Converter10/RConn1 -- Ideal Torque Source RL/RConn1
  Simulink-PS Converter12/RConn1 -- Ideal Torque Source FL/RConn1
  Tire (Simple) RL/RConn1 -- Tire-Road Interaction (Magic Formula) RL/LConn2
  Simulink-PS Converter11/RConn1 -- Ideal Torque Source FR/RConn1
  Belt Drive FR/LConn1 -- Ideal Torque Source FR/LConn1
  Belt Drive RL/LConn1 -- Ideal Torque Source RL/LConn1
  Mechanical Rotational Reference3/LConn1 -- Ideal Torque Source FR/RConn2
  Belt Drive RR/RConn1 -- Tire (Simple) RR/LConn1
  Belt Drive FL/RConn1 -- Tire (Simple) FL/LConn1
  Mechanical Rotational Reference1/LConn1 -- Ideal Torque Source RR/RConn2
  v_lin1/LConn1 -- Vehicle Body/LConn2
  Belt Drive RL/RConn1 -- Tire (Simple) RL/LConn1
  Tire (Simple) FR/RConn1 -- Tire-Road Interaction (Magic Formula) FR/LConn2
  Vehicle Body/RConn3 -- Simulink-PS Converter8/RConn1
  Mechanical Rotational Reference8/LConn1 -- Ideal Torque Source FL/RConn2
  Simulink-PS Converter3/RConn1 -- Vehicle Body/LConn3
  Tire (Simple) RR/RConn1 -- Tire-Road Interaction (Magic Formula) RR/LConn2
  Tire (Simple) FL/RConn1 -- Tire-Road Interaction (Magic Formula) FL/LConn2
  Mechanical Rotational Reference2/LConn1 -- Ideal Torque Source RL/RConn2
  Belt Drive RR/LConn1 -- Ideal Torque Source RR/LConn1
  Belt Drive FL/LConn1 -- Ideal Torque Source FL/LConn1
  Tire-Road Interaction (Magic Formula) RR/RConn1 -- PS-Simulink Converter/LConn1
  PS-Simulink Converter1/LConn1 -- Tire-Road Interaction (Magic Formula) RL/RConn1
  PS-Simulink Converter3/LConn1 -- Tire-Road Interaction (Magic Formula) FR/RConn1
  PS-Simulink Converter4/LConn1 -- Tire-Road Interaction (Magic Formula) FL/RConn1
